simulink model "Model_f_simulink_f_20"  (R2015b)
settings: Solver=VariableStepAuto  StartTime=0.0  StopTime=3  FixedStep=0.001  RelTol=0.5e-3
undefined symbols (not defined in the file): ADAMS_cwd, ADAMS_exec, ADAMS_host, ADAMS_init, ADAMS_inputs, ADAMS_outputs, ADAMS_prefix, ADAMS_static, ADAMS_sysdir
libraries: simulink x2
settings Model: Creator=Ali  LastModifiedBy=Ali

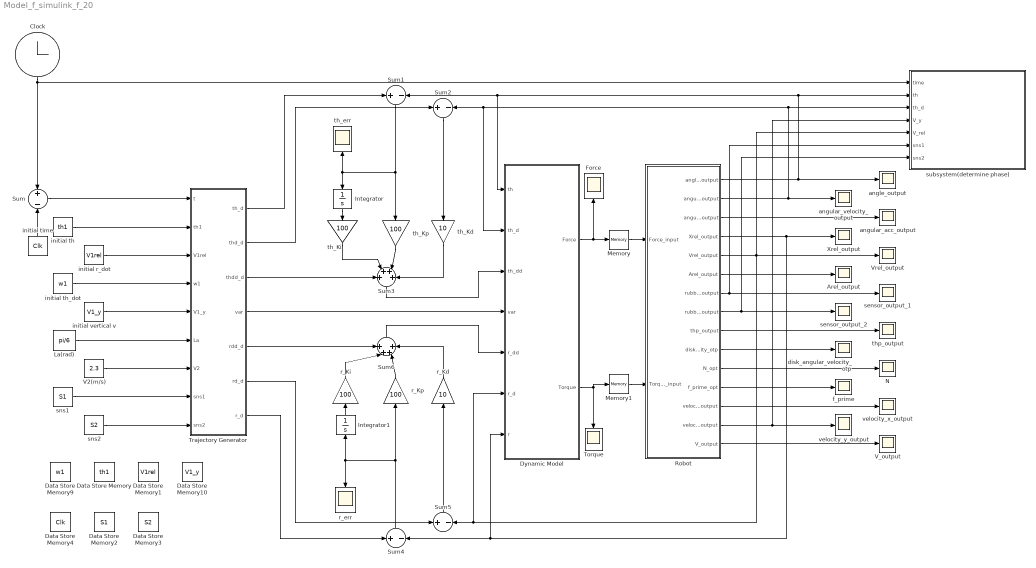
== system Model_f_simulink_f_20 ==
  Arel_output : Scope
  Clock : Clock
  Data Store Memory : DataStoreMemory  DataStoreName=th1
  Data Store Memory1 : DataStoreMemory  DataStoreName=V1rel
  Data Store Memory10 : DataStoreMemory  DataStoreName=V1_y
  Data Store Memory2 : DataStoreMemory  DataStoreName=S1
  Data Store Memory3 : DataStoreMemory  DataStoreName=S2
  Data Store Memory4 : DataStoreMemory  DataStoreName=Clk
  Data Store Memory9 : DataStoreMemory  DataStoreName=w1
  Dynamic Model : MATLAB Function  TreatAsAtomicUnit=on
  Force : Scope
  Integrator : Integrator
  Integrator1 : Integrator
  La(rad) : Constant  Value=pi/6
  Memory : Memory
  Memory1 : Memory
  N : Scope
  Robot : Subsystem
  Sum{,1..2,4..5} (5 alike) : Sum  Inputs=+-
  Sum3 : Sum  Inputs=++++
  Sum6 : Sum  Inputs=++++
  Torque : Scope
  Trajectory Generator : MATLAB Function  TreatAsAtomicUnit=on
  V2(m/s) : Constant  Value=2.3
  V_output : Scope
  Vrel_output : Scope
  Xrel_output : Scope
  angle_output : Scope
  angular_acc_output : Scope
  angular_velocity_output : Scope
  disk_angular_velocity_otp : Scope
  f_prime : Scope
  initial r_dot : DataStoreRead  DataStoreName=V1rel
  initial th : DataStoreRead  DataStoreName=th1
  initial th_dot : DataStoreRead  DataStoreName=w1
  initial time : DataStoreRead  DataStoreName=Clk
  initial vertical v : DataStoreRead  DataStoreName=V1_y
  r_Kd : Gain  Gain=10
  r_Ki : Gain  Gain=100
  r_Kp : Gain  Gain=100
  r_err : Scope
  sensor_output_1 : Scope
  sensor_output_2 : Scope
  sns1 : DataStoreRead  DataStoreName=S1
  sns2 : DataStoreRead  DataStoreName=S2
  subsystem(determine phase) : Subsystem  TreatAsAtomicUnit=on
  th_Kd : Gain  Gain=10
  th_Ki : Gain  Gain=100
  th_Kp : Gain  Gain=100
  th_err : Scope
  thp_output : Scope
  velocity_x_output : Scope
  "velocity_y_output      " : Scope
  wires:
  Clock/1 -> Sum/1, subsystem(determine phase)/1(time)
  initial time/1 -> Sum/2
  Robot/3("angular_acc_output ") -> angular_acc_output/1
  Robot/6("Arel_output ") -> Arel_output/1
  Robot/10(disk_angular_velocity_otp) -> disk_angular_velocity_otp/1
  Robot/11(N_opt) -> N/1
  Robot/13(velocity_x_output) -> velocity_x_output/1
  Robot/14(velocity_y_output) -> subsystem(determine phase)/4(V_y), "velocity_y_output      "/1
  Robot/15("V_output ") -> V_output/1
  Robot/9(thp_output) -> thp_output/1
  Robot/7(rubber_1_sensor_output) -> subsystem(determine phase)/6(sns1), sensor_output_1/1
  Robot/8(rubber_2_sensor_output) -> subsystem(determine phase)/7(sns2), sensor_output_2/1
  Trajectory Generator/4(var) -> Dynamic Model/4(var)
  V2(m/s)/1 -> Trajectory Generator/7(V2)
  La(rad)/1 -> Trajectory Generator/6(La)
  initial vertical v/1 -> Trajectory Generator/5(V1_y)
  initial th_dot/1 -> Trajectory Generator/4(w1)
  initial r_dot/1 -> Trajectory Generator/3(V1rel)
  sns1/1 -> Trajectory Generator/8(sns1)
  sns2/1 -> Trajectory Generator/9(sns2)
  initial th/1 -> Trajectory Generator/2(th1)
  Dynamic Model/1(Force) -> Force/1, Memory/1
  Dynamic Model/2(Torque) -> Torque/1, Memory1/1
  Sum/1 -> Trajectory Generator/1(t)
  Robot/12("f_prime_opt ") -> f_prime/1
  Trajectory Generator/1(th_d) -> Sum1/1
  Sum1/1 -> th_err/1, Integrator/1, th_Kp/1
  Sum2/1 -> th_Kd/1
  Trajectory Generator/2(thd_d) -> Sum2/1
  th_Kp/1 -> Sum3/3
  Trajectory Generator/3(thdd_d) -> Sum3/1
  th_Kd/1 -> Sum3/4
  Sum3/1 -> Dynamic Model/3(th_dd)
  r_Kp/1 -> Sum6/3
  Sum6/1 -> Dynamic Model/5(r_dd)
  Trajectory Generator/5(rdd_d) -> Sum6/1
  Trajectory Generator/7(r_d) -> Sum4/1
  Sum4/1 -> r_Kp/1, r_err/1, Integrator1/1
  Trajectory Generator/6(rd_d) -> Sum5/1
  Sum5/1 -> r_Kd/1
  r_Kd/1 -> Sum6/4
  Memory/1 -> Robot/1("Force_input ")
  Memory1/1 -> Robot/2(Torque_input)
  Robot/4("Xrel_output ") -> Sum4/2, Dynamic Model/7(r), Xrel_output/1
  Robot/5(Vrel_output) -> Vrel_output/1, Dynamic Model/6(r_d), Sum5/2, subsystem(determine phase)/5(V_rel)
  Robot/2(angular_velocity_output) -> subsystem(determine phase)/3(th_d), Sum2/2, Dynamic Model/2(th_d), angular_velocity_output/1
  Robot/1("angle_output ") -> subsystem(determine phase)/2(th), Sum1/2, Dynamic Model/1(th), angle_output/1
  Integrator/1 -> th_Ki/1
  Integrator1/1 -> r_Ki/1
  th_Ki/1 -> Sum3/2
  r_Ki/1 -> Sum6/2

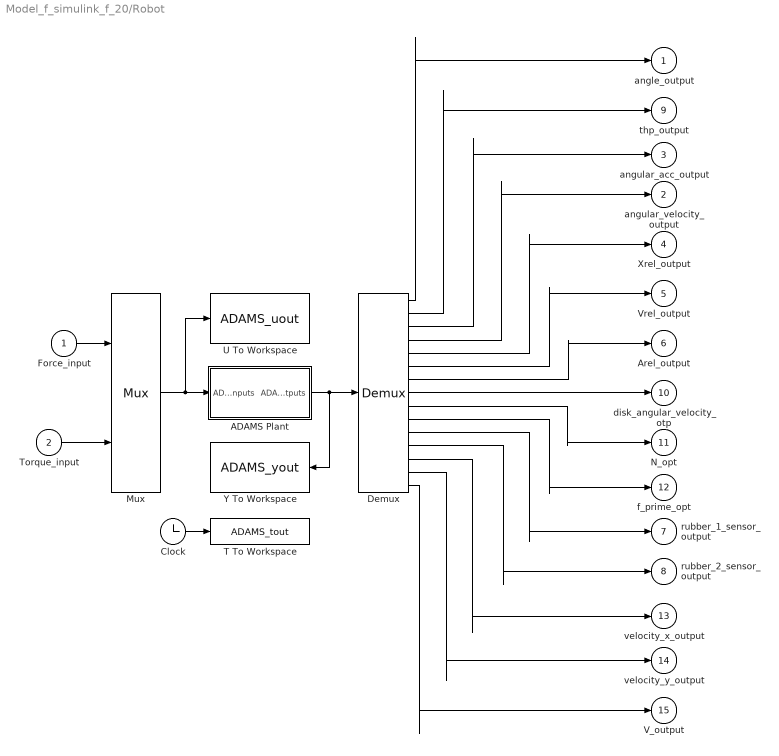
== system Model_f_simulink_f_20/Robot ==
  "Force_input " : Inport
  Torque_input : Inport  Port=2
  ADAMS Plant : Subsystem  LoadFcn=|  InitFcn=clear mex  mask(Adams Plant){exevie=ADAMS_sysdir, nam_in=ADAMS_inputs, namout=ADAMS_outputs, nampre=ADAMS_prefix, outfil='mytest_20', exesol=ADAMS_exec, stat=ADAMS_static, inicmd=[ADAMS_init], exetyp=C++, comtyp=PIPE(DDE), workdir=ADAMS_cwd, ada_host=ADAMS_host, modani=interactive, modsim=discrete, dft=no, simulink_lead_cosim=yes, pin_interp_order=0, pout_extrap_order=0, pin_extrap_order=0, pout_interp_order=0, dt_out=0.001, o_rate=1, more=off}
      | %check based on dialog box setting for when setting by popup menu                                             
      | if exist('ADAMS_solver_type')                                                                                 
      |   if strcmp(ADAMS_solver_type,'C++')                                                                          
      |     set_param(gcb,'exetyp','C++');                                                                            
      |   else                                                                                                        
      |     set_param(gcb,'exetyp','Fortran');                                                                        
      |   end                                                                                                         
      | else                                                                                                          
      |   set_param(gcb,'exetyp','C++');                                                                              
      | end                                                                                                           
      | %set the mode if using acar_solver                                                                            
      | %REQUIRED HERE BECAUSE BELOW CAUSES MDLTERMINATE TO BE CALLED 2 TIMES IN MIDDLE OF SIMULATION WHEN SET IN MASK
      |                                                                                                               
      | %enable the direct feedthrough, sim mode, anim mode parameters by default                                     
      |                                                                                                               
      | if exist('set_some_params_states')                                                                            
      |                                                                                                               
      |   set_some_params_states({'dft','modsim','modani'},{'on','on','on'},'MaskEnables',gcb)                        
      |   %turn on direct feedthrough option                                                                          
      |   set_some_params_states({'dft'},{'on'},'MaskVisibilities',gcb)                                               
      |                                                                                                               
      |  end                                                                                                          
      |                                                                                                               
      |                                                                                                               
      | if exist('ADAMS_exec')                                                                                        
      |   if and(strcmp(get_param(gcb,'exesol'),'ADAMS_exec'),strcmp(ADAMS_exec,'acar_solver'))                       
      |     %set the sim mode to discrete -- only supported mode                                                      
      |     set_param(gcb,'modsim','discrete')                                                                        
      |      %turn off direct feedthrough option                                                                      
      |      set_some_params_states({'dft'},{'off'},'MaskVisibilities',gcb)                                           
      |     %set the animation mode to batch -- only supported mode                                                   
      |     set_param(gcb,'modani','batch')                                                                           
      |     %disable the direct feedthrough, sim mode, anim mode parameters                                           
      |     set_some_params_states({'modsim','modani'},{'off','off'},'MaskEnables',gcb)                               
      |   end                                                                                                         
      | end
      mask prompts: exevie "Adams install directory"; nam_in "Adams/View input names"; namout "Adams/View output names"; nampre "Adams model file prefix"; outfil "Output files prefix (opt.: if blank - no output)"; exesol "User executable (opt.: if blank - use standard)"; stat "Initial static simulation flag"; inicmd "Initialization commands"; exetyp "Adams/Solver type"; comtyp "Interprocess option"; workdir "Adams working directory"; ada_host "Adams host"; modani "Animation mode"; modsim "Simulation mode"; dft "Direct feedthrough"; simulink_lead_cosim "Discrete Computational Order - Simulink Leads Adams"; pin_interp_order "Plant input interpolation order"; pout_extrap_order "Plant output extrapolation order"; pin_extrap_order "Plant input extrapolation order"; pout_interp_order "Plant output interpolation order"; dt_out "Communication interval"; o_rate "Number of communications per output step"; more "More parameters"
      mask help: Simulate any Adams plant model either in Adams/Solver form (.adm file) or in Adams/View form (.cmd file)
      settings: OpenFcn=|
      | open_system(gcb,'mask')
      | if not(exist('set_some_params_states'))
      | 
      | warning('The script "set_some_params_states.m" cannot be found in the MATLAB PATH.  Cannot update the ADAMS Plant S-Function parameters.')
      | 
      | warning('Recommended action(optional):  run the Adams/Controls .m file first to help choose the correct settings in the Adams S-Function block.')
      | 
      | end
      mask Help:
      | <html>
      | This S-Function represents the non-linear Adams Plant with the inputs sent to the Adams model <br>
      |  and the outputs generated by the Adams model.  See the Adams/Controls documentation for more <br>
      | information.  This plant uses the following variables:<br>
      | <br>
      | <b>ADAMS_sysdir  :</b> Adams installation directory<br>
      | <b>ADAMS_inputs  :</b> Input variables View names vector<br>
      | <b>ADAMS_outputs :</b> Outputs variables View names vector<br>
      | <b>ADAMS_prefix  : </b>ADAMS model files prefix (.adm, .cmd); also doubles as output files prefix<br>
      | <b>ADAMS_exec :</b> Adams/Solver user library or keyword (e.g., acar_solver)<br>
      | <b>ADAMS_static :</b> yes|no - initial static before Co-simulation(discrete)/Function Evaluation(continuous)<br>
      | <b>ADAMS_init :</b>Initialization commands (i.e., Adams/View or Solver commands, depending on setting for Animation mode)<br>
      | <b>ADAMS_cwd : </b> Current working directory (for TCP/IP)<br>
      | <b>ADAMS_host : </b>Name of Adams server host (for TCP/IP)<br>
      | <b>ADAMS_mode :</b> Linear or non-linear (i.e., co-sim, function eval)<br>
      | <b>ADAMS_solver_type :</b>Fortran or C++ (used to set popup menu when first loaded) <br>
      | 
      | 
      | <br>
      | The following settings can be chosen:<br>
      | <br>
      | <b>Adams/Solver type:</b>  Fortran or C++ (will also set ADAMS_solver_type)<br>
      | <b>Interprocess option:</b> Pipe(DDE) or TCP/IP; TCP/IP can allow different machines run Adams and MATLAB<br>
      | <b>Animation mode:</b> batch (Solver, uses .adm) or interactive (View, uses .cmd)<br>
      | <b>Simulation mode:</b> discrete (Co-simulation) or continuous (Function Evaluation)<br>
      | <b>Discrete Computational Order - Simulink Lead Adams:</b> for discrete mode, chooses if Simulink leads the integration (yes) or lags (no);<br> if set to "no", can remove algebraic loop<br>
      | <b>Plant input interpolation order:</b> 0 = zero-order hold; 1 = linear (discrete mode only, where Simulink leads)<br>
      | <b>Plant output extrapolation order:</b> 0 = zero-order hold;1 = linear(discrete mode only, where Simulink leads)<br>
      | <b>Plant input extrapolation order:</b> 0 = zero-order hold; 1 = linear (discrete mode only, where Adams leads)<br>
      | <b>Plant output interpolation order:</b> 0 = zero-order hold;1 = linear(discrete mode only, where Adams leads)<br>
      | <b>Direct feedthrough:</b> yes|no - yes = Input directly effect output(continuous mode-only)<br>
      | <b>Communication interval:</b> Time step at which Co-simulation exchange information (e.g.,0.005); also controls <br>output for continuous mode (Function Evaluation)<br>
      | <b>Number of communications per output step: </b>Sets Adams output rate (.res, .req, .gra) integer value (default: 1)<br>
      | </html>
      mask Callback exesol:
      | if exist('set_some_params_states')
      | %enable the direct feedthrough, sim mode, anim mode parameters
      | set_some_params_states({'dft','modsim','modani'},{'on','on','on'},'MaskEnables',gcb)
      | %turn on direct feedthrough option
      | set_some_params_states({'dft'},{'on'},'MaskVisibilities',gcb)
      | end
      | 
      | if exist('ADAMS_exec')
      |   if and(strcmp(get_param(gcb,'exesol'),'ADAMS_exec'),strcmp(ADAMS_exec,'acar_solver'))
      |     %set the sim mode to discrete -- only supported mode
      |     %REMOVED:  BELOW CAUSES MDLTERMINATE TO BE CALLED 2 TIMES IN MIDDLE OF SIMULATION
      |     %Now in LoadFcn callback
      |     %set_param(gcb,'modsim','discrete')
      |      %turn off direct feedthrough option
      |     set_some_params_states({'dft'},{'off'},'MaskVisibilities',gcb)
      |     %set the animation mode to batch -- only supported mode
      |     %REMOVED:  BELOW CAUSES MDLTERMINATE TO BE CALLED 2 TIMES IN MIDDLE OF SIMULATION
      |     %Now in LoadFcn callback
      |     %set_param(gcb,'modani','batch')
      |     %disable the direct feedthrough, sim mode, anim mode parameters
      |     set_some_params_states({'modsim','modani'},{'off','off'},'MaskEnables',gcb)
      |   end
      | end
      mask TypeOptions exetyp: Fortran | C++
      mask Callback exetyp:
      | if strcmp(get_param(gcb,'exetyp'),'C++')
      |     ADAMS_solver_type='C++';
      | else
      |     ADAMS_solver_type='Fortran';
      | end
      mask TypeOptions comtyp: PIPE(DDE) | TCP/IP
      mask Callback comtyp:
      | if exist('set_some_params_states')
      | if strcmp(get_param(gcb,'comtyp'),'PIPE(DDE)')
      |     %turn off cwd, host options
      |     set_some_params_states({'ada_host','workdir'},{'off','off'},'MaskVisibilities',gcb)
      | else%if strcmp(get_param(gcb,'modsim'),'TCP/IP')
      |     %turn on cwd, host options
      |     set_some_params_states({'ada_host','workdir'},{'on','on'},'MaskVisibilities',gcb)
      | end
      | end
      mask TypeOptions modani: batch | interactive
      mask TypeOptions modsim: discrete | continuous
      mask Callback modsim:
      | if exist('set_some_params_states')
      | if strcmp(get_param(gcb,'modsim'),'discrete')
      |      %turn off direct feedthrough option
      |     set_some_params_states({'dft'},{'off'},'MaskVisibilities',gcb)
      |     %turn on discrete co-sim type if want to see more
      |     if strcmp(get_param(gcb,'more'),'on')
      |         set_some_params_states({'simulink_lead_cosim'},{'on'},'MaskVisibilities',gcb)
      |     end
      |     if strcmp(get_param(gcb,'simulink_lead_cosim'),'yes')
      |         %turn on interpolation/extrapolation options
      |         set_some_params_states({'pin_interp_order','pout_extrap_order',},{'on','on'},'MaskVisibilities',gcb)
      |     else
      |         set_some_params_states({'pin_extrap_order','pout_interp_order'},{'on','on'},'MaskVisibilities',gcb)
      |     end
      | else%if strcmp(get_param(gcb,'modsim'),'continuous')
      |      %turn off direct feedthrough option
      |     set_some_params_states({'dft'},{'on'},'MaskVisibilities',gcb)
      |     %turn off interpolation/extrapolation options
      |     set_some_params_states({'pin_interp_order','pout_extrap_order','pin_extrap_order','pout_interp_order','simulink_lead_cosim'},{'off','off','off','off','off'},'MaskVisibilities',gcb)
      | end
      | end
      mask TypeOptions dft: no | yes
      mask TypeOptions simulink_lead_cosim: yes | no
      mask Callback simulink_lead_cosim:
      | if exist('set_some_params_states')
      | if (strcmp(get_param(gcb,'simulink_lead_cosim'),'yes') && strcmp(get_param(gcb,'modsim'),'discrete'))
      |      %turn off unused interpolate/extrapolate options
      |     set_some_params_states({'pin_extrap_order','pout_interp_order'},{'off','off'},'MaskVisibilities',gcb)
      |     %turn on used interpolate/extrapolate options
      |     set_some_params_states({'pin_interp_order','pout_extrap_order'},{'on','on'},'MaskVisibilities',gcb)
      | elseif (strcmp(get_param(gcb,'simulink_lead_cosim'),'no') && strcmp(get_param(gcb,'modsim'),'discrete'))
      |     %turn on used interpolate/extrapolate options
      |     set_some_params_states({'pin_extrap_order','pout_interp_order'},{'on','on'},'MaskVisibilities',gcb)
      |      %turn off unused interpolate/extrapolate options
      |     set_some_params_states({'pin_interp_order','pout_extrap_order'},{'off','off'},'MaskVisibilities',gcb)
      | end
      | end
      mask TypeOptions pin_interp_order: 0 | 1
      mask TypeOptions pout_extrap_order: 0 | 1
      mask TypeOptions pin_extrap_order: 0 | 1
      mask TypeOptions pout_interp_order: 0 | 1
      mask Callback more:
      | if exist('set_some_params_states')
      | if (strcmp(get_param(gcb,'more'),'on'))
      |      %turn on infrequently used options
      |     set_some_params_states({'exevie','nam_in','namout','exesol','stat','inicmd'},{'on','on','on','on','on','on'},'MaskVisibilities',gcb)
      |     if strcmp(get_param(gcb,'modsim'),'discrete')
      |         set_some_params_states({'simulink_lead_cosim'},{'on'},'MaskVisibilities',gcb)
      |     end
      | elseif (strcmp(get_param(gcb,'more'),'off'))
      |     %turn off infrequently used options
      |     set_some_params_states({'exevie','nam_in','namout','exesol','stat','inicmd'},{'off','off','off','off','off','off'},'MaskVisibilities',gcb)
      |     if strcmp(get_param(gcb,'modsim'),'discrete')
      |         set_some_params_states({'simulink_lead_cosim'},{'off'},'MaskVisibilities',gcb)
      |     end
      | end
      | end
      mask Display: disp( 'MSC Software' )
  Clock : Clock
  Demux : Demux  Outputs=15
  Mux : Mux  Inputs=2
  T To Workspace : ToWorkspace  VariableName=ADAMS_tout
      settings: MaxDataPoints=100000
  U To Workspace : ToWorkspace  VariableName=ADAMS_uout
      settings: MaxDataPoints=100000
  Y To Workspace : ToWorkspace  VariableName=ADAMS_yout
      settings: MaxDataPoints=100000
  "angle_output " : Outport
  angular_velocity_output : Outport  Port=2
  "angular_acc_output " : Outport  Port=3
  "Xrel_output " : Outport  Port=4
  Vrel_output : Outport  Port=5
  "Arel_output " : Outport  Port=6
  rubber_1_sensor_output : Outport  Port=7
  rubber_2_sensor_output : Outport  Port=8
  thp_output : Outport  Port=9
  disk_angular_velocity_otp : Outport  Port=10
  N_opt : Outport  Port=11
  "f_prime_opt " : Outport  Port=12
  velocity_x_output : Outport  Port=13
  velocity_y_output : Outport  Port=14
  "V_output " : Outport  Port=15
  wires:
  Clock/1 -> T To Workspace/1
  Mux/1 -> ADAMS Plant/1(ADAMS inputs), U To Workspace/1
  ADAMS Plant/1(ADAMS outputs) -> Demux/1, Y To Workspace/1
  Demux/1 -> "angle_output "/1
  Demux/2 -> thp_output/1
  Demux/3 -> "angular_acc_output "/1
  Demux/4 -> angular_velocity_output/1
  Demux/5 -> "Xrel_output "/1
  Demux/6 -> Vrel_output/1
  Demux/7 -> "Arel_output "/1
  Demux/8 -> disk_angular_velocity_otp/1
  Demux/9 -> N_opt/1
  Demux/10 -> "f_prime_opt "/1
  Demux/11 -> rubber_1_sensor_output/1
  Demux/12 -> rubber_2_sensor_output/1
  Demux/13 -> velocity_x_output/1
  Demux/14 -> velocity_y_output/1
  Demux/15 -> "V_output "/1
  "Force_input "/1 -> Mux/1
  Torque_input/1 -> Mux/2

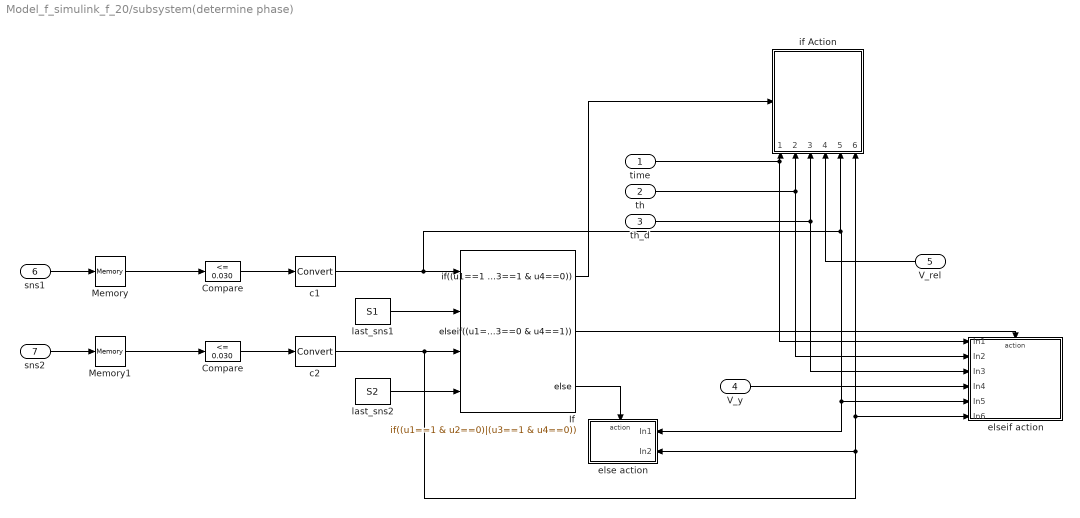
== system Model_f_simulink_f_20/subsystem(determine phase) ==
  time : Inport
  th : Inport  Port=2
  th_d : Inport  Port=3
  V_y : Inport  Port=4
  V_rel : Inport  Port=5
  sns1 : Inport  Port=6
  sns2 : Inport  Port=7
  Compare : simulink/Logic and Bit Operations/Compare To Constant  relop=<=  const=0.030  OutDataTypeStr=uint8
  "Compare " : simulink/Logic and Bit Operations/Compare To Constant  relop=<=  const=0.030  OutDataTypeStr=uint8
  If : If  NumInputs=4  IfExpression=(u1==1 & u2==0)|(u3==1 & u4==0)  ElseIfExpressions=(u1==0 & u2==1)|(u3==0 & u4==1)
  Memory : Memory
  Memory1 : Memory
  c1 : DataTypeConversion
  c2 : DataTypeConversion
  else action : Subsystem  TreatAsAtomicUnit=on
  elseif action : Subsystem  TreatAsAtomicUnit=on
  if Action : Subsystem  TreatAsAtomicUnit=on
  last_sns1 : DataStoreRead  DataStoreName=S1
  last_sns2 : DataStoreRead  DataStoreName=S2
  wires:
  th/1 -> if Action/2(In2), elseif action/2(In2)
  th_d/1 -> if Action/3(In3), elseif action/3(In3)
  V_y/1 -> elseif action/4(In4)
  V_rel/1 -> if Action/4(In4)
  time/1 -> elseif action/1(In1), if Action/1(In1)
  c1/1 -> If/1, else action/1(In1), elseif action/5(In5), if Action/5(In5)
  last_sns1/1 -> If/2
  If/3 -> else action/Action
  c2/1 -> if Action/6(In6), elseif action/6(In6), else action/2(In2), If/3
  last_sns2/1 -> If/4
  If/1 -> if Action/Action
  "Compare "/1 -> c1/1
  Compare/1 -> c2/1
  If/2 -> elseif action/Action
  sns1/1 -> Memory/1
  sns2/1 -> Memory1/1
  Memory/1 -> "Compare "/1
  Memory1/1 -> Compare/1

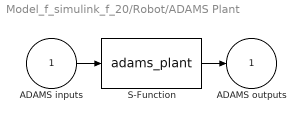
== system Model_f_simulink_f_20/Robot/ADAMS Plant ==
  ADAMS inputs : Inport
  S-Function : S-Function  StopFcn=clear mex  FunctionName=adams_plant  Parameters=exevie,exesol,stat,outfil,nampre,o_rate,nam_in,namout,dft,modsim,modani,dt_out,inicmd,exetyp,comtyp,ada_host, workdir,pin_interp_order,pout_extrap_order,pin_extrap_order,pout_interp_order,simulink_lead_cosim  SFunctionDeploymentMode=off  EnableBusSupport=off
  ADAMS outputs : Outport  InitialOutput=0
  wires:
  ADAMS inputs/1 -> S-Function/1
  S-Function/1 -> ADAMS outputs/1

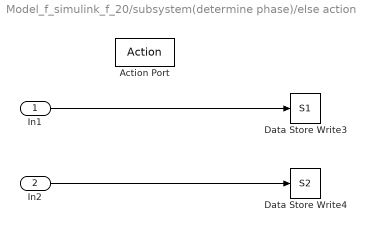
== system Model_f_simulink_f_20/subsystem(determine phase)/else action ==
  In1 : Inport
  In2 : Inport  Port=2
  Action Port : ActionPort  ActionType=else
  Data Store Write3 : DataStoreWrite  DataStoreName=S1
  Data Store Write4 : DataStoreWrite  DataStoreName=S2
  wires:
  In1/1 -> Data Store Write3/1
  In2/1 -> Data Store Write4/1

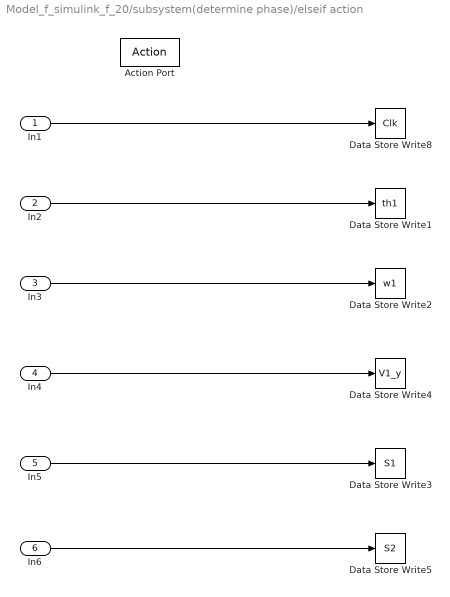
== system Model_f_simulink_f_20/subsystem(determine phase)/elseif action ==
  In1 : Inport
  In2 : Inport  Port=2
  In3 : Inport  Port=3
  In4 : Inport  Port=4
  In5 : Inport  Port=5
  In6 : Inport  Port=6
  Action Port : ActionPort  ActionType=elseif
  Data Store Write1 : DataStoreWrite  DataStoreName=th1
  Data Store Write2 : DataStoreWrite  DataStoreName=w1
  Data Store Write3 : DataStoreWrite  DataStoreName=S1
  Data Store Write4 : DataStoreWrite  DataStoreName=V1_y
  Data Store Write5 : DataStoreWrite  DataStoreName=S2
  Data Store Write8 : DataStoreWrite  DataStoreName=Clk
  wires:
  In5/1 -> Data Store Write3/1
  In2/1 -> Data Store Write1/1
  In3/1 -> Data Store Write2/1
  In1/1 -> Data Store Write8/1
  In4/1 -> Data Store Write4/1
  In6/1 -> Data Store Write5/1

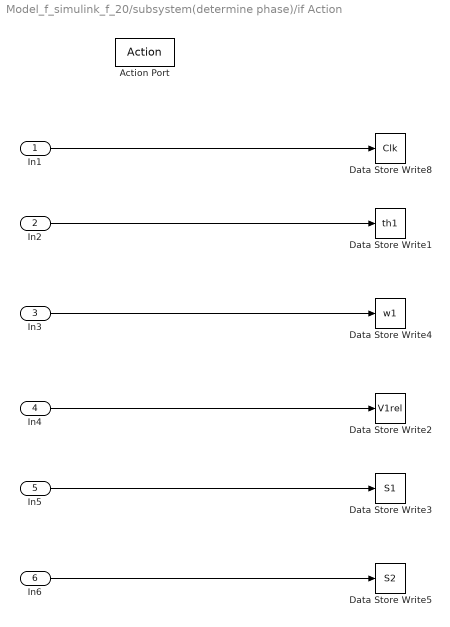
== system Model_f_simulink_f_20/subsystem(determine phase)/if Action ==
  In1 : Inport
  In2 : Inport  Port=2
  In3 : Inport  Port=3
  In4 : Inport  Port=4
  In5 : Inport  Port=5
  In6 : Inport  Port=6
  Action Port : ActionPort  ActionType=then
  Data Store Write1 : DataStoreWrite  DataStoreName=th1
  Data Store Write2 : DataStoreWrite  DataStoreName=V1rel
  Data Store Write3 : DataStoreWrite  DataStoreName=S1
  Data Store Write4 : DataStoreWrite  DataStoreName=w1
  Data Store Write5 : DataStoreWrite  DataStoreName=S2
  Data Store Write8 : DataStoreWrite  DataStoreName=Clk
  wires:
  In1/1 -> Data Store Write8/1
  In2/1 -> Data Store Write1/1
  In4/1 -> Data Store Write2/1
  In5/1 -> Data Store Write3/1
  In3/1 -> Data Store Write4/1
  In6/1 -> Data Store Write5/1

== matlab function Model_f_simulink_f_20/Trajectory Generator ==
  data: t input; th_d output; th1 input; V1rel input; w1 input; V1_y input; thd_d output; La input; V2 input; sns1 input; sns2 input; thdd_d output; var output; rdd_d output; rd_d output; r_d output
function [ th_d,thd_d,thdd_d,var,rdd_d,rd_d,r_d ] = fcn1(t,th1,V1rel,w1,V1_y,La,V2,sns1,sns2)
R=0.307+.02;            %center of mass +0.02 = maximum positive deformation of spring(delta x)
th_d=0.0; thd_d=0.0; thdd_d=0.0; r_d=0.06; rd_d=0.0; rdd_d=0.0; var=0;
T=0.11;                 %stance time
x2=0.09;                %spring maximum length
L0=0.06;                %spring free length
Ga=(2*R+T*pi-((2*R+T*pi)^2-4*T*(2*R*La+T*(pi^2/4-2)))^0.5)/2/T;
w2=V2*(La-Ga)/T;        %desired th_dot
th2=T*w2/V2;            %desired th
if (sns1==1 || sns2==1) 
    V2rel=V2*cos(Ga);       %desired r_dot 
    V1rel=-abs(V1rel);      %intial r_dot
    if (t>T) 
       var=0;
    else
        if (th1<0.001 && th1>-0.001); w1=0;  end
        %th trajectory(cubic spline)---------
        B1=th1;
        B2=w1;
        B3=3*(th2-th1)/T^2-2*w1/T-w2/T;
        B4=2*(th1-th2)/T^3+w1/T^2+w2/T^2;

        thl=[B4 B3 B2 B1];
        thl_d=polyder(thl);
        thl_dd=polyder(thl_d);
        th_d=polyval(thl,t);
        thd_d=polyval(thl_d,t);
        thdd_d=polyval(thl_dd,t);
        %r trajectory(cubic spline)----------
        A1=L0;
        A2=V1rel;
        A3=3*(x2-L0)/T^2-(2*V1rel+V2rel)/T;
        A4=2*(L0-x2)/T^3+(V1rel+V2rel)/T^2;      

        x=[A4 A3 A2 A1];
        x_d=polyder(x);
        x_dd=polyder(x_d);
        r_d=polyval(x,t);
        rd_d=polyval(x_d,t);
        rdd_d=polyval(x_dd,t);

        if (sns1==1); var=1; end
        if (sns2==1); var=2; r_d=2*L0-r_d; rd_d=-rd_d; rdd_d=-rdd_d; end
    end
end

if (sns1==0 && sns2==0)
    if (th1<0.001 && th1>-0.001)
        var=0;
    else
        g=9.8;                   %gravity
        T=2*abs(V1_y)/g+0.015;   %flight time
        th2=pi-th2;       %desired th
        %th trajectory(cubic spline)---------
        B1=th1;
        B2=w1;
        B3=3*(th2-th1)/T^2-2*w1/T-w2/T;
        B4=2*(th1-th2)/T^3+w1/T^2+w2/T^2;

        thl=[B4 B3 B2 B1];
        thl_d=polyder(thl);
        thl_dd=polyder(thl_d);
        th_d=polyval(thl,t);
        if (th_d>1.5813); th_d=th_d-pi; end 
        thd_d=polyval(thl_d,t);
        thdd_d=polyval(thl_dd,t);

        var=3;
    end
end

end

== matlab function Model_f_simulink_f_20/Dynamic Model ==
  data: th input; th_d input; th_dd input; var input; r_dd input; r_d input; r input; Force output; Torque output
function [ Force,Torque ] = fcn2(th,th_d,th_dd,var,r_dd,r_d,r)
    
    g=9.8;              %gravity
    Il=0.0196;          %link's moment of inertia
    mtot=2.365;         %total mass
    mbar=0.00712;       %bar mass
    L0=0.06;            %spring free length
    c=37;               %damping coeff
    k=400;              %spring stiffness coeff
    Force=0; Torque=0;
    if (var==1)                                                         %--sensor 1 touches ground
        R=.307+r-L0;                                                    %radius of center of mass
        Force=(mtot*(r_dd-th_d*th_d*R)+k*(r-L0)+mtot*g*cos(th)+c*r_d);  %linear moror force
        f_prime=mtot*(R*th_dd+2*th_d*r_d)-mtot*g*sin(th);               %normal-to-the-link reaction ground force
        N=Force+mbar*g*cos(th)+k*(L0-r)-c*r_d-mbar*R*th_d*th_d;         %parallel-with-the-link reaction ground force
        Torque=Il*th_dd+f_prime*R+N*0.03*sin(th);                       %angular moror torque
    end
    if (var==2)                                                         %--sensor 2 touches ground
        r=2*L0-r; r_d=-r_d; r_dd=-r_dd;    
        R=.307+r-L0;                                                    %radius of center of mass
        Force=-(mtot*(r_dd-th_d*th_d*R)+k*(r-L0)+mtot*g*cos(th)+c*r_d); %linear moror force
        f_prime=mtot*(R*th_dd+2*th_d*r_d)-mtot*g*sin(th);               %normal-to-the-link reaction ground force
        N=-Force+mbar*g*cos(th)+k*(L0-r)-c*r_d-mbar*R*th_d*th_d;        %parallel-with-the-link reaction ground force
        Torque=Il*th_dd+f_prime*R+N*0.03*sin(th);                       %angular moror torque
    end
    if (var==3)                                                         %--flight phase
        Torque=Il*th_dd;                                                %angular moror torque
        Force=0;
    end
end
